simulink model "TestDebitMoteurNew"  (R2024b)
settings: Solver=FixedStepDiscrete  StartTime=0.0  StopTime=SimuPumpStop  FixedStep=0.1  RelTol=1e-6  EnableMultiTasking=on
undefined symbols (not defined in the file): nv_remp, Pamb, PcolTest, PumpedTest, Rair, RegimeTest, Tamb, TempsTest, TimePumpedTest, Vcyl
settings Model: Creator=a030141  LastModifiedBy=ramse
settings SolverCC: AlgebraicLoopSolver=TrustRegion
settings DataIOCC: LimitDataPoints=on  SaveFormat=Array  SignalLoggingSaveFormat=ModelDataLogs  ReturnWorkspaceOutputs=off  SignalLoggingName=sigsOut
settings OptimizationCC: InitFltsAndDblsToZero=on  LifeSpan=inf
settings DebuggingCC: SaveWithParameterizedLinksMsg=none  UnderspecifiedInitializationDetection=Classic  MergeDetectMultiDrivingBlocksExec=none  SignalResolutionControl=TryResolveAllWithWarning  MultiTaskDSMMsg=warning  MultiTaskCondExecSysMsg=none  FcnCallInpInsideContextMsg=warning  UnconnectedInputMsg=warning  UnconnectedOutputMsg=warning  UnconnectedLineMsg=warning  SFUnexpectedBacktrackingDiag=warning  SFNoUnconditionalDefaultTransitionDiag=warning  SFExecutionAtInitializationDiag=none  ArithmeticOperatorsInVariantConditions=warning
settings HardwareCC: ProdBitPerPointer=32  ProdBitPerSizeT=32  ProdBitPerPtrDiffT=32  ProdLargestAtomicFloat=None  ProdIntDivRoundTo=Undefined  ProdEndianess=Unspecified  ProdWordSize=32  ProdHWDeviceType=32-bit Generic  TargetUnknown=on
settings ModelReferenceCC: PropagateSignalLabelsOutOfModel=off
settings RTWCC: GPUComputeCapability=3.5
settings CodeAppCC: StateflowObjectComments=on
settings GRTTargetCC: TargetFcnLib=ansi_tfl_tmw.mat  TargetLangStandard=C89/C90 (ANSI)  CombineOutputUpdateFcns=off  GRTInterface=on
settings ConfigComp: CovMetricSettings=dw  CovSaveCumulativeToWorkspaceVar=on  CovSaveSingleToWorkspaceVar=on

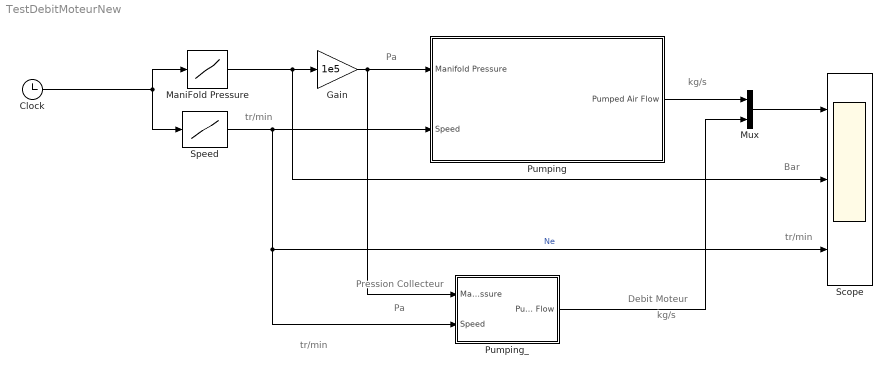
== system TestDebitMoteurNew ==
  note: Pression Collecteur
  note: Debit Moteur
  note: kg/s
  note: Pa
  note: Bar
  note: tr/min
  note: tr/min
  note: Pa
  note: tr/min
  note: kg/s
  Clock : Clock
  Gain : Gain  Gain=1e5  SaturateOnIntegerOverflow=on  OutDataTypeStr=Inherit: Same as input  ParamDataTypeStr=Inherit: Same as input
  ManiFold Pressure : Lookup  InputValues=TempsTest  Table=PcolTest
  Mux : Mux  Inputs=2
  Pumping : Subsystem
  Pumping_ : Subsystem
  Scope : Scope  NumInputPorts=3
  Speed : Lookup  InputValues=TempsTest  Table=RegimeTest
  wires:
  Clock/1 -> ManiFold Pressure/1, Speed/1
  ManiFold Pressure/1 -> Gain/1, Scope/2
  Mux/1 -> Scope/1
  Pumping/1(Pumped Air Flow) -> Mux/1
  Gain/1 -> Pumping_/1(Manifold Pressure), Pumping/1(Manifold Pressure)
  Speed/1 -> Pumping_/2(Speed), Scope/3, Pumping/2(Speed)  "Ne"
  Pumping_/1(Pumped Air Flow) -> Mux/2

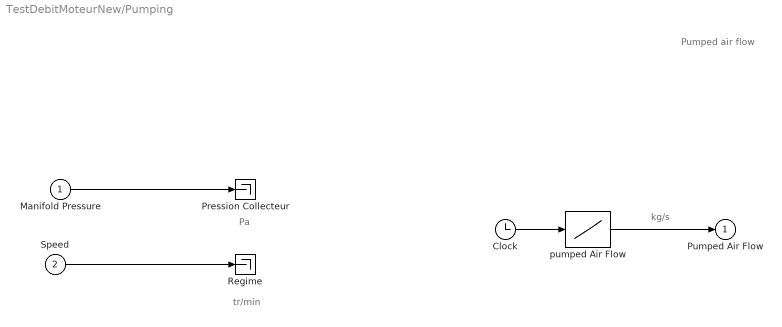
== system TestDebitMoteurNew/Pumping ==
  note: Pumped air flow
  note: kg/s
  note: Pa
  note: tr/min
  Manifold Pressure : Inport
  Speed : Inport  Port=2
  Clock : Clock
  Pression Collecteur : Terminator
  Regime : Terminator
  pumped Air Flow : Lookup  InputValues=TimePumpedTest  Table=PumpedTest
  Pumped Air Flow : Outport
  wires:
  Manifold Pressure/1 -> Pression Collecteur/1
  Speed/1 -> Regime/1
  pumped Air Flow/1 -> Pumped Air Flow/1
  Clock/1 -> pumped Air Flow/1

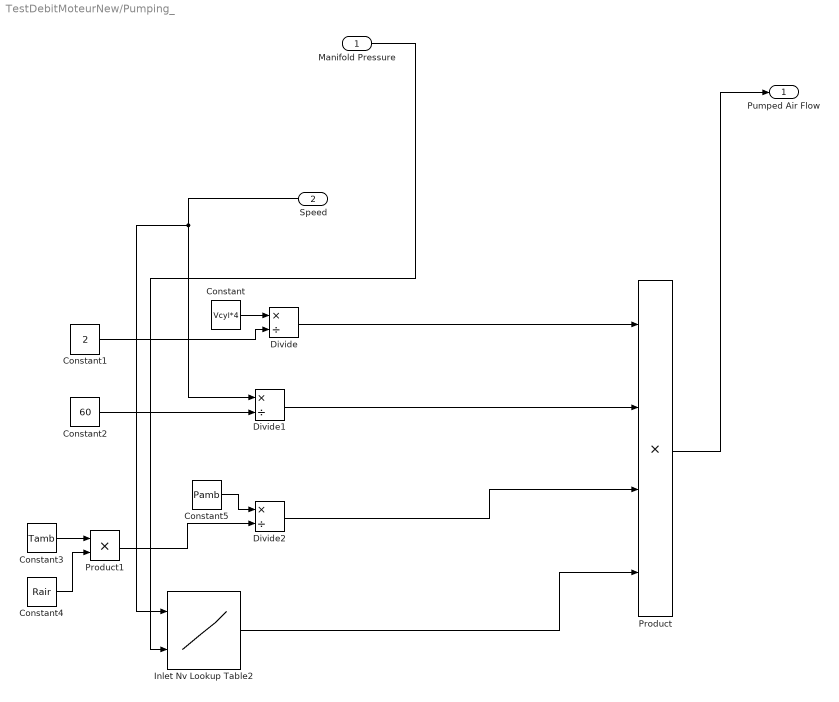
== system TestDebitMoteurNew/Pumping_ ==
  Manifold Pressure : Inport
  Speed : Inport  Port=2
  Constant : Constant  Value=Vcyl*4
  Constant1 : Constant  Value=2
  Constant2 : Constant  Value=60
  Constant3 : Constant  Value=Tamb
  Constant4 : Constant  Value=Rair
  Constant5 : Constant  Value=Pamb
  Divide : Product  Inputs=*/
  Divide1 : Product  Inputs=*/
  Divide2 : Product  Inputs=*/
  Inlet Nv Lookup Table2 : Lookup2D  RowIndex=Ne_remp  ColumnIndex=Pcol_remp  Table=nv_remp
  Product : Product  Inputs=4
  Product1 : Product
  Pumped Air Flow : Outport
  wires:
  Constant3/1 -> Product1/1
  Constant5/1 -> Divide2/1
  Divide/1 -> Product/1
  Constant/1 -> Divide/1
  Divide2/1 -> Product/3
  Divide1/1 -> Product/2
  Product1/1 -> Divide2/2
  Inlet Nv Lookup Table2/1 -> Product/4
  Constant1/1 -> Divide/2
  Constant2/1 -> Divide1/2
  Constant4/1 -> Product1/2
  Product/1 -> Pumped Air Flow/1
  Speed/1 -> Inlet Nv Lookup Table2/1, Divide1/1
  Manifold Pressure/1 -> Inlet Nv Lookup Table2/2
